simulink model "main"  (Simulink 7.5)
settings: Solver=ode45  StartTime=0.0  StopTime=1  RelTol=1e-3
InitFcn:
  | Ts=50e-6;
  | fs=5e3;
  | freq=60;
libraries: powerlib x21, simulink x4, powerlib_extras x1
settings Model: Creator=AnandG  LastModifiedBy=New  CovModelRefEnable=off
settings DataIOCC: LimitDataPoints=off  SaveFormat=StructureWithTime
settings OptimizationCC: ExpressionDepthLimit=128
settings DebuggingCC: UnderspecifiedInitializationDetection=Simplified  MergeDetectMultiDrivingBlocksExec=error  SolverPrmCheckMsg=none  FcnCallInpInsideContextMsg=Enable All  StateNameClashWarn=none
settings HardwareCC: ProdIntDivRoundTo=Zero  ProdEndianess=LittleEndian  ProdHWDeviceType=Specified
settings CodeAppCC: CustomSymbolStrType=$N$R$M_T
settings GRTTargetCC: TargetFunctionLibrary=C89/C90 (ANSI)

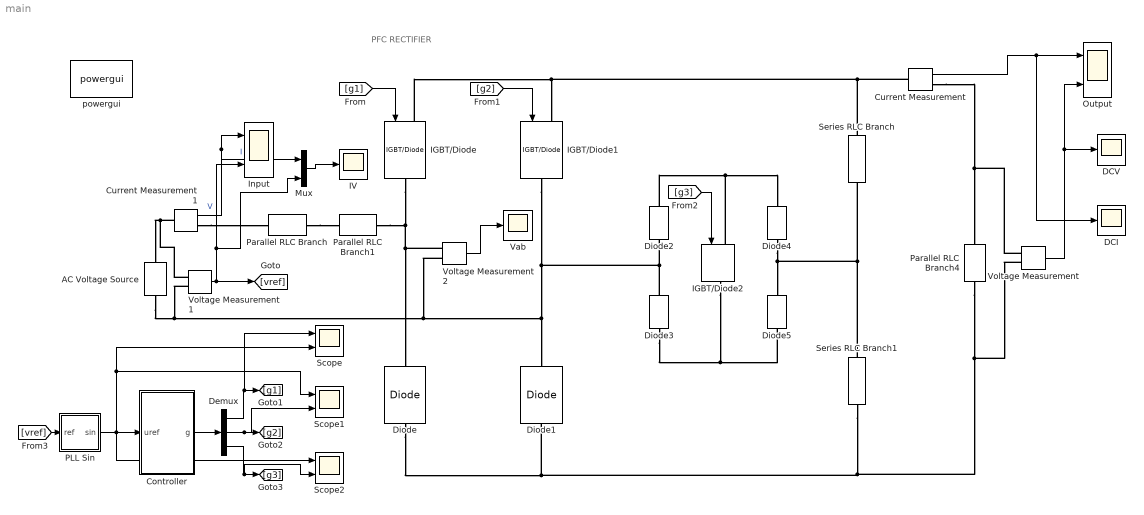
== system main ==
  note: PFC RECTIFIER
  AC Voltage Source : powerlib/Electrical Sources/AC Voltage Source  DialogController=POWERSYS.PowerSysDialog  SystemSampleTime=-1  Amplitude=200  Phase=0  Frequency=freq  SampleTime=0  Measurements=None
  Controller : Subsystem
  Current Measurement : powerlib/Measurements/Current Measurement  DialogController=POWERSYS.PowerSysDialog  SystemSampleTime=-1  PhasorSimulation=off  OutputType=Complex  PSBequivalent=0
  Current Measurement1 : powerlib/Measurements/Current Measurement  DialogController=POWERSYS.PowerSysDialog  SystemSampleTime=-1  PhasorSimulation=off  OutputType=Complex  PSBequivalent=0
  DCI : Scope
      settings: YMin=-0.45508  YMax=4.09541  SaveName=ScopeData10
  DCV : Scope
      settings: YMin=-36.40671  YMax=327.63308  SaveName=ScopeData9
  Demux : Demux  Outputs=3
  Diode{,1..5} (6 alike) : powerlib/Power Electronics/Diode  DialogController=POWERSYS.PowerSysDialog  SystemSampleTime=-1  Ron=0.001  Lon=0  Vf=0.8  IC=0  UseSnubber=off  Rs=500  Cs=250e-9  Measurements=off
  IGBT/Diode : powerlib/Power Electronics/IGBT//Diode  DialogController=POWERSYS.PowerSysDialog  SystemSampleTime=-1  Ron=1e-3  Rs=1e5  Cs=inf  Measurements=off
  IGBT/Diode1 : powerlib/Power Electronics/IGBT//Diode  DialogController=POWERSYS.PowerSysDialog  SystemSampleTime=-1  Ron=1e-3  Rs=1e5  Cs=inf  Measurements=off
  IGBT/Diode2 : powerlib/Power Electronics/IGBT//Diode  DialogController=POWERSYS.PowerSysDialog  SystemSampleTime=-1  Ron=1e-3  Rs=1e5  Cs=inf  Measurements=off
  IV : Scope
      settings: YMin=-346.4025  YMax=299.99485  SaveName=ScopeData12
  Input : Scope  NumInputPorts=2
      settings: YMin=-97.24613~-5  YMax=53.35628~5
  Mux : Mux  Inputs=2
  Output : Scope  NumInputPorts=2
      settings: TimeRange=1  YMin=-36.40671~-5  YMax=327.63308~5
  PLL Sin : Subsystem
  Parallel RLC Branch : powerlib/Elements/Parallel RLC Branch  DialogController=POWERSYS.PowerSysDialog  PhysicalDomain=powersysdomain  SubClassName=unknown  LeftPortType=p1  RightPortType=p1  LConnTagsString=a  RConnTagsString=__new0  BranchType=L  Resistance=1  Inductance=2.5e-3  SetiL0=off  InitialCurrent=0  Capacitance=1e-6  Setx0=off  InitialVoltage=0  Measurements=None
  Parallel RLC Branch1 : powerlib/Elements/Parallel RLC Branch  DialogController=POWERSYS.PowerSysDialog  PhysicalDomain=powersysdomain  SubClassName=unknown  LeftPortType=p1  RightPortType=p1  LConnTagsString=a  RConnTagsString=__new0  BranchType=R  Resistance=1  Inductance=1e-3  SetiL0=off  InitialCurrent=0  Capacitance=1e-6  Setx0=off  InitialVoltage=0  Measurements=None
  Parallel RLC Branch4 : powerlib/Elements/Parallel RLC Branch  DialogController=POWERSYS.PowerSysDialog  PhysicalDomain=powersysdomain  SubClassName=unknown  LeftPortType=p1  RightPortType=p1  LConnTagsString=a  RConnTagsString=__new0  BranchType=R  Resistance=80  Inductance=1e-3  SetiL0=off  InitialCurrent=0  Capacitance=1e-6  Setx0=off  InitialVoltage=0  Measurements=None
  Scope : Scope  NumInputPorts=2
      settings: YMin=-1.25~-5  YMax=1.25~5  SaveName=ScopeData2
  Scope1 : Scope  NumInputPorts=2
      settings: YMin=-1.25~-5  YMax=1.25~5  SaveName=ScopeData3
  Scope2 : Scope  NumInputPorts=2
      settings: YMin=-1.25~-5  YMax=1.25~5  SaveName=ScopeData4
  Series RLC Branch : powerlib/Elements/Series RLC Branch  DialogController=POWERSYS.PowerSysDialog  PhysicalDomain=powersysdomain  SubClassName=unknown  LeftPortType=p1  RightPortType=p1  LConnTagsString=__new0  RConnTagsString=__new0  BranchType=C  Resistance=1  Inductance=1e-3  SetiL0=off  InitialCurrent=0  Capacitance=1000e-6  Setx0=off  InitialVoltage=0  Measurements=None
  Series RLC Branch1 : powerlib/Elements/Series RLC Branch  DialogController=POWERSYS.PowerSysDialog  PhysicalDomain=powersysdomain  SubClassName=unknown  LeftPortType=p1  RightPortType=p1  LConnTagsString=__new0  RConnTagsString=__new0  BranchType=C  Resistance=1  Inductance=1e-3  SetiL0=off  InitialCurrent=0  Capacitance=1000e-6  Setx0=off  InitialVoltage=0  Measurements=None
  Vab : Scope
      settings: YMin=-346.4025  YMax=299.99485  SaveName=ScopeData8
  Voltage Measurement : powerlib/Measurements/Voltage Measurement  DialogController=POWERSYS.PowerSysDialog  SystemSampleTime=-1  PhasorSimulation=off  OutputType=Complex  PSBequivalent=0
  Voltage Measurement1 : powerlib/Measurements/Voltage Measurement  DialogController=POWERSYS.PowerSysDialog  SystemSampleTime=-1  PhasorSimulation=off  OutputType=Complex  PSBequivalent=0
  Voltage Measurement2 : powerlib/Measurements/Voltage Measurement  DialogController=POWERSYS.PowerSysDialog  SystemSampleTime=-1  PhasorSimulation=off  OutputType=Complex  PSBequivalent=0
  powergui : powerlib/powergui  Priority=1  SystemSampleTime=-1  SimulationMode=Discrete  SampleTime=Ts  frequency=60  SPID=off  DisableSnubberDevices=off  DisableRonSwitches=off  DisableVfSwitches=off  SwTol=0  Interpol=off  frequencyindice=60  echomessages=off  HookPort=off  DisplayEquations=off  FunctionMessages=off  EnableUseOfTLC=off  x0status=blocks  RestoreLinks=warning  ResistiveCurrentMeasurement=off  Frange=[0:2:500]  Ylog=off  Xlog=on  ShowGrid=off  save=off  variable=ZData  structure=0  ZoomFFT=off  StartTime=0.0  cycles=1  DisplayStyle=1  fundamental=60  FreqAxis=off  MaxFrequency=1000  frequencyindicesteady=1  RmsSteady=1  display=off  Ts=0  methode=off
  wires:
  Current Measurement1/1 -> Input/1, Mux/1  "I"
  Voltage Measurement1/1 -> [vref], Input/2, Mux/2  "V"
  Current Measurement/1 -> DCI/1, Output/1
  Voltage Measurement/1 -> DCV/1, Output/2
  [g1] -> IGBT/Diode/1
  [g2] -> IGBT/Diode1/1
  [g3] -> IGBT/Diode2/1
  Controller/1(g) -> Demux/1
  Demux/1 -> Scope/1, [g1]
  Demux/2 -> Scope1/2, [g2]
  Demux/3 -> Scope2/2, [g3]
  [vref] -> PLL Sin/1(ref)
  PLL Sin/1(sin) -> Scope2/1, Scope1/1, Scope/2, Controller/1(uref)
  Voltage Measurement2/1 -> Vab/1
  Mux/1 -> IV/1
  connections:
  IGBT/Diode/RConn1 -- Voltage Measurement2/LConn1 -- Diode/RConn1 -- Parallel RLC Branch1/RConn1
  Diode3/RConn1 -- Voltage Measurement2/LConn2 -- AC Voltage Source/LConn1 -- Voltage Measurement1/LConn2 -- Diode1/RConn1 -- IGBT/Diode1/RConn1 -- Diode2/LConn1
  Diode/LConn1 -- Series RLC Branch1/RConn1 -- Parallel RLC Branch4/RConn1 -- Voltage Measurement/LConn2 -- Diode1/LConn1
  IGBT/Diode/LConn1 -- Series RLC Branch/LConn1 -- Current Measurement/LConn1 -- IGBT/Diode1/LConn1
  Series RLC Branch1/LConn1 -- Diode5/RConn1 -- Diode4/LConn1 -- Series RLC Branch/RConn1
  Parallel RLC Branch/RConn1 -- Parallel RLC Branch1/LConn1
  Current Measurement/RConn1 -- Parallel RLC Branch4/LConn1 -- Voltage Measurement/LConn1
  Current Measurement1/LConn1 -- Voltage Measurement1/LConn1 -- AC Voltage Source/RConn1
  Current Measurement1/RConn1 -- Parallel RLC Branch/LConn1
  IGBT/Diode2/LConn1 -- Diode2/RConn1 -- Diode4/RConn1
  IGBT/Diode2/RConn1 -- Diode5/LConn1 -- Diode3/LConn1

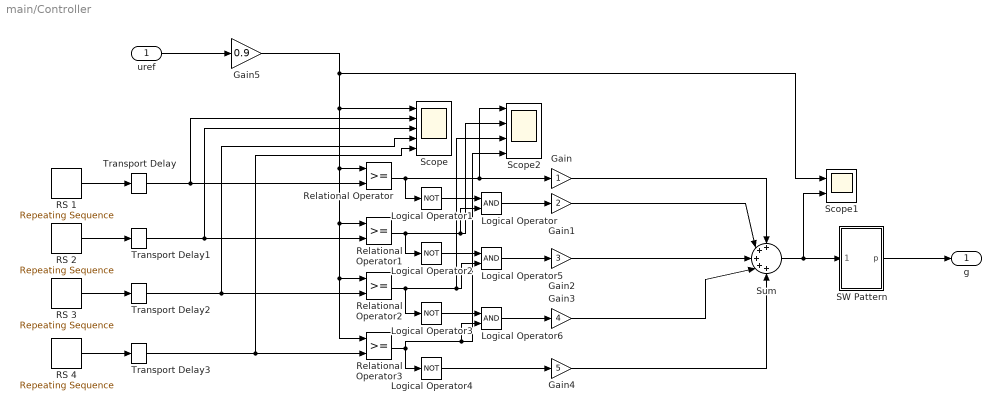
== system main/Controller ==
  uref : Inport
  Gain : Gain
  Gain1 : Gain  Gain=2
  Gain2 : Gain  Gain=3
  Gain3 : Gain  Gain=4
  Gain4 : Gain  Gain=5
  Gain5 : Gain  Gain=0.9
  Logical Operator : Logic  AllPortsSameDT=off  OutDataTypeMode=boolean  OutDataTypeStr=boolean
  Logical Operator{1..4} (4 alike) : Logic  Operator=NOT  AllPortsSameDT=off  OutDataTypeMode=boolean  OutDataTypeStr=boolean
  Logical Operator5 : Logic  AllPortsSameDT=off  OutDataTypeMode=boolean  OutDataTypeStr=boolean
  Logical Operator6 : Logic  AllPortsSameDT=off  OutDataTypeMode=boolean  OutDataTypeStr=boolean
  RS 1 : simulink/Sources/Repeating Sequence  SystemSampleTime=-1  rep_seq_t="[0 (1/(fs*4))*1  (1/(fs*4))*2  (1/(fs*4))*3  (1/(fs*4))*4]"  rep_seq_y=[0.5 1 0.5 1 0.5]
  RS 2 : simulink/Sources/Repeating Sequence  SystemSampleTime=-1  rep_seq_t="[0 (1/(fs*4))*1  (1/(fs*4))*2  (1/(fs*4))*3  (1/(fs*4))*4]"  rep_seq_y=[0 0.5 0 0.5 0]
  RS 3 : simulink/Sources/Repeating Sequence  SystemSampleTime=-1  rep_seq_t="[0 (1/(fs*4))*1  (1/(fs*4))*2  (1/(fs*4))*3  (1/(fs*4))*4]"  rep_seq_y=[-0.5 0 -0.5 0 -0.5]
  RS 4 : simulink/Sources/Repeating Sequence  SystemSampleTime=-1  rep_seq_t="[0 (1/(fs*4))*1  (1/(fs*4))*2  (1/(fs*4))*3  (1/(fs*4))*4]"  rep_seq_y=[-1 -0.5 -1 -0.5 -1]
  Relational Operator{,1..3} (4 alike) : RelationalOperator  LogicOutDataTypeMode=boolean  OutDataTypeStr=boolean  ZeroCross=off
  SW Pattern : Subsystem
  Scope : Scope  NumInputPorts=5
      settings: YMin=-1.32133~-5~-5~-5~-5  YMax=1.29563~5~5~5~5  SaveName=ScopeData5
  Scope1 : Scope  NumInputPorts=2
      settings: YMin=-1.75~-5  YMax=5.75~5  SaveName=ScopeData6
  Scope2 : Scope  NumInputPorts=4
      settings: YMin=-0.125~-5~-5~-5  YMax=1.125~5~5~5  SaveName=ScopeData7
  Sum : Sum  Inputs=5
  Transport Delay{,1..3} (4 alike) : TransportDelay  DelayTime=(1/(fs*8))*1
  g : Outport
  wires:
  Relational Operator2/1 -> Scope2/3, Logical Operator5/2, Logical Operator3/1
  SW Pattern/1(p) -> g/1
  Relational Operator1/1 -> Scope2/2, Logical Operator/2, Logical Operator2/1
  Relational Operator/1 -> Gain/1, Scope2/1, Logical Operator1/1
  Sum/1 -> Scope1/2, SW Pattern/1(state)
  RS 2/1 -> Transport Delay1/1
  Logical Operator3/1 -> Logical Operator6/1
  RS 1/1 -> Transport Delay/1
  Logical Operator1/1 -> Logical Operator/1
  RS 3/1 -> Transport Delay2/1
  RS 4/1 -> Transport Delay3/1
  Logical Operator2/1 -> Logical Operator5/1
  Relational Operator3/1 -> Scope2/4, Logical Operator6/2, Logical Operator4/1
  Logical Operator/1 -> Gain1/1
  Logical Operator5/1 -> Gain2/1
  Logical Operator6/1 -> Gain3/1
  Logical Operator4/1 -> Gain4/1
  Gain/1 -> Sum/1
  Gain1/1 -> Sum/2
  Gain2/1 -> Sum/3
  Gain3/1 -> Sum/4
  Gain4/1 -> Sum/5
  uref/1 -> Gain5/1
  Gain5/1 -> Scope1/1, Relational Operator3/1, Relational Operator2/1, Relational Operator1/1, Relational Operator/1, Scope/1
  Transport Delay/1 -> Relational Operator/2, Scope/2
  Transport Delay1/1 -> Relational Operator1/2, Scope/3
  Transport Delay2/1 -> Relational Operator2/2, Scope/4
  Transport Delay3/1 -> Relational Operator3/2, Scope/5

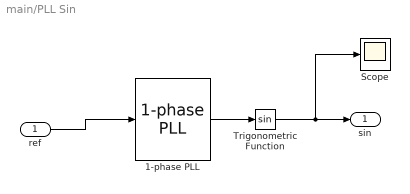
== system main/PLL Sin ==
  ref : Inport
  1-phase PLL : powerlib_extras/Control  Blocks/1-phase PLL  DialogController=POWERSYS.PowerSysDialog  SystemSampleTime=-1  Par_Init=[0 freq]  ParK=[ 180 3200 1 ]  AGC=off
  Scope : Scope
      settings: SaveName=ScopeData11
  Trigonometric Function : Trigonometry
  sin : Outport
  wires:
  Trigonometric Function/1 -> sin/1, Scope/1
  1-phase PLL/2 -> Trigonometric Function/1
  ref/1 -> 1-phase PLL/1

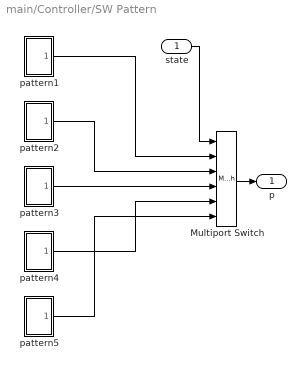
== system main/Controller/SW Pattern ==
  state : Inport
  Multiport Switch : MultiPortSwitch  Inputs=5  zeroidx=off
  pattern1 : Subsystem
  pattern2 : Subsystem
  pattern3 : Subsystem
  pattern4 : Subsystem
  pattern5 : Subsystem
  p : Outport
  wires:
  pattern3/1(gate) -> Multiport Switch/4
  pattern2/1(gate) -> Multiport Switch/3
  pattern4/1(gate) -> Multiport Switch/5
  pattern5/1(gate) -> Multiport Switch/6
  state/1 -> Multiport Switch/1
  Multiport Switch/1 -> p/1
  pattern1/1(gate) -> Multiport Switch/2

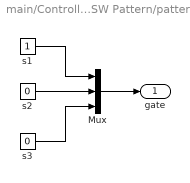
== system main/Controller/SW Pattern/pattern1 ==
  Mux : Mux  Inputs=3
  s1 : Constant
  s2 : Constant  Value=0
  s3 : Constant  Value=0
  gate : Outport
  wires:
  Mux/1 -> gate/1
  s3/1 -> Mux/3
  s2/1 -> Mux/2
  s1/1 -> Mux/1

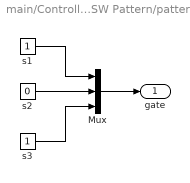
== system main/Controller/SW Pattern/pattern2 ==
  Mux : Mux  Inputs=3
  s1 : Constant
  s2 : Constant  Value=0
  s3 : Constant
  gate : Outport
  wires:
  Mux/1 -> gate/1
  s3/1 -> Mux/3
  s2/1 -> Mux/2
  s1/1 -> Mux/1

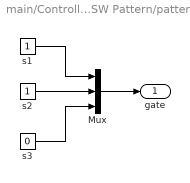
== system main/Controller/SW Pattern/pattern3 ==
  Mux : Mux  Inputs=3
  s1 : Constant
  s2 : Constant
  s3 : Constant  Value=0
  gate : Outport
  wires:
  Mux/1 -> gate/1
  s3/1 -> Mux/3
  s2/1 -> Mux/2
  s1/1 -> Mux/1

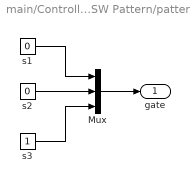
== system main/Controller/SW Pattern/pattern4 ==
  Mux : Mux  Inputs=3
  s1 : Constant  Value=0
  s2 : Constant  Value=0
  s3 : Constant
  gate : Outport
  wires:
  Mux/1 -> gate/1
  s3/1 -> Mux/3
  s2/1 -> Mux/2
  s1/1 -> Mux/1

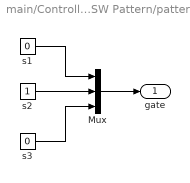
== system main/Controller/SW Pattern/pattern5 ==
  Mux : Mux  Inputs=3
  s1 : Constant  Value=0
  s2 : Constant
  s3 : Constant  Value=0
  gate : Outport
  wires:
  Mux/1 -> gate/1
  s3/1 -> Mux/3
  s2/1 -> Mux/2
  s1/1 -> Mux/1
